simulink model "Example_A_Simulink"  (R2024b)
settings: Solver=VariableStepAuto  StartTime=0.0  StopTime=10.0  RelTol=1e-3
settings Model: Creator=user  LastModifiedBy=user

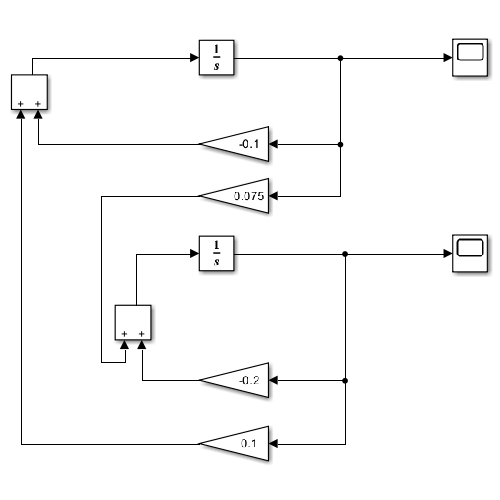
[thumbnail: Simulink's stored preview of the top-level diagram]
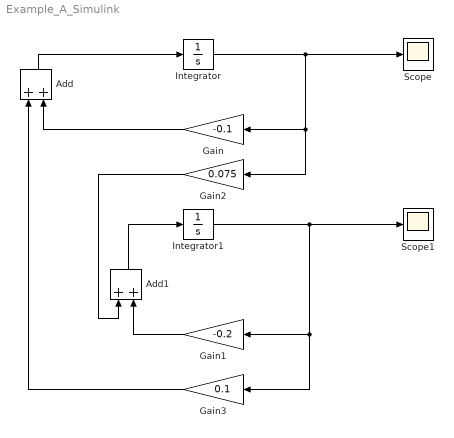
== system Example_A_Simulink ==
  Add : Sum
  Add1 : Sum
  Gain : Gain  Gain=-0.1
  Gain1 : Gain  Gain=-0.2
  Gain2 : Gain  Gain=0.075
  Gain3 : Gain  Gain=0.1
  Integrator : Integrator  InitialCondition=-17
  Integrator1 : Integrator  InitialCondition=-21
  Scope : Scope
  Scope1 : Scope
  wires:
  Add/1 -> Integrator/1
  Gain/1 -> Add/2
  Integrator/1 -> Scope/1, Gain2/1, Gain/1
  Add1/1 -> Integrator1/1
  Integrator1/1 -> Scope1/1, Gain3/1, Gain1/1
  Gain1/1 -> Add1/2
  Gain2/1 -> Add1/1
  Gain3/1 -> Add/1
